simulink model "AttAndOrbitPropagator"  (R2017a)
settings: Solver=FixedStepAuto  StartTime=0.0  StopTime=24*3600  FixedStep=10  RelTol=1e-3  EnableMultiTasking=on
PreLoadFcn:
  | InitialiseJ2
values from neighbouring files (symbols this model uses):
  a = (mu/(n*2*pi/(24*3600))^2)^(1/3)    [InitialiseJ2.m]
  e = L3(1,5)/1e7    [InitialiseJ2.m]
  h = (mu*rp*(1 + e))^0.5    [InitialiseJ2.m]
  i = L3(1,3)    [InitialiseJ2.m]
  J2 = 0.0010836    [InitialiseJ2.m]
  mu = 398600.4415    [InitialiseJ2.m]
  omega = L3(1,6)    [InitialiseJ2.m]
  R_earth = 6378.137    [InitialiseJ2.m]
  RAAN = L3(1,4)    [InitialiseJ2.m]
  T = 2*pi*sqrt(a^3/mu)    [InitialiseJ2.m]
  t0 = M/(2*pi)*T    [InitialiseJ2.m]
libraries: sharedtransform x4, vrlib x3
settings Model: PauseTimes=0  NumberOfSteps=10  SnapshotBufferSize=10000  SnapshotInterval=1  Creator="TEAM  STUDSAT -2"  LastModifiedBy=Navaneet
settings OptimizationCC: LifeSpan=inf
settings DebuggingCC: SFUnexpectedBacktrackingDiag=warning  SFNoUnconditionalDefaultTransitionDiag=warning  SFExecutionAtInitializationDiag=none
settings GRTTargetCC: TargetLangStandard=C89/C90 (ANSI)  GeneratePreprocessorConditionals=Disable all
settings ConfigComp: CovMetricSettings=dw  CovHtmlReporting=on  CovSaveCumulativeToWorkspaceVar=on  CovSaveSingleToWorkspaceVar=on  CovExternalEMLEnable=off

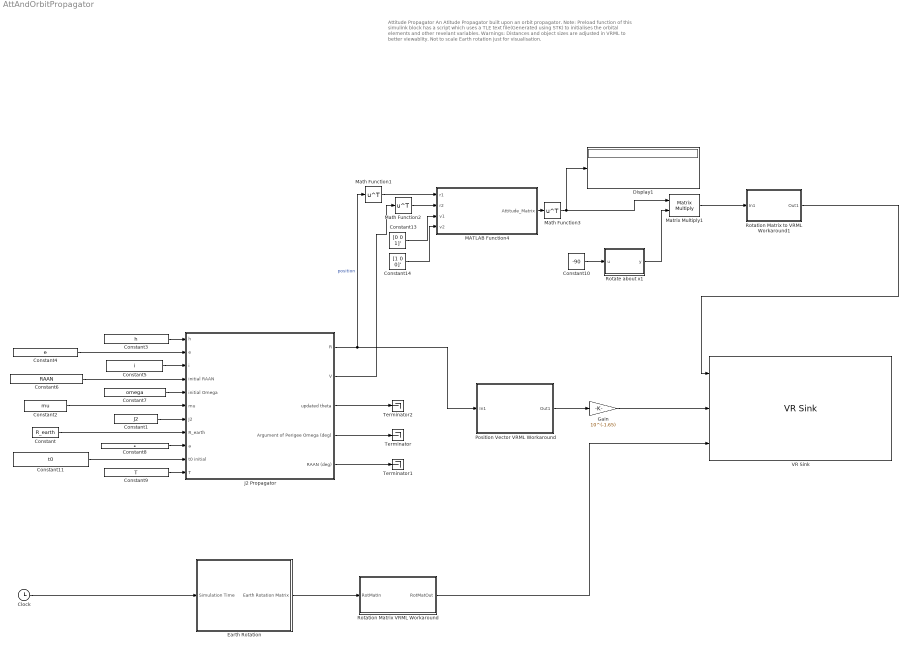
== system AttAndOrbitPropagator ==
  note: Attitude Propagator
      | An Atitude Propagator built upon an orbit propagator.
      |
      | Note:
      | Preload function of this simulink block has a script which uses a TLE text file(Generated using STK) to initialises the orbital elements and other revelant variables.
      |
      | Warnings:
      | Distances and object sizes are adjusted in VRML to better viewablity. Not to scale
      | Earth rotation just for visualisation.
  Clock : Clock
  Constant : Constant  Value=R_earth
  Constant1 : Constant  Value=J2
  Constant10 : Constant  Value=-90
  Constant11 : Constant  Value=t0
  Constant13 : Constant  Value=[0 0 1]'  VectorParams1D=off
  Constant14 : Constant  Value=[1 0 0]'  VectorParams1D=off
  Constant2 : Constant  Value=mu
  Constant3 : Constant  Value=h
  Constant4 : Constant  Value=e
  Constant5 : Constant  Value=i
  Constant6 : Constant  Value=RAAN
  Constant7 : Constant  Value=omega
  Constant8 : Constant  Value=a
  Constant9 : Constant  Value=T
  Display1 : Display
  Earth Rotation : Subsystem
  Gain : Gain  Gain=10^(-1.65)
  J2 Propagator : Subsystem
  MATLAB Function4 : MATLAB Function  TreatAsAtomicUnit=on
  Math Function1 : Math  Operator=transpose  SaturateOnIntegerOverflow=on
  Math Function2 : Math  Operator=transpose  SaturateOnIntegerOverflow=on
  Math Function3 : Math  Operator=transpose  SaturateOnIntegerOverflow=on
  Matrix Multiply1 : Product  Multiplication=Matrix(*)
  Position Vector VRML Workaround : Subsystem
  Rotate about x1 : MATLAB Function  TreatAsAtomicUnit=on
  Rotation Matrix VRML Workaround : Subsystem
  Rotation Matrix to VRML Workaround1 : Subsystem
  Terminator : Terminator
  Terminator1 : Terminator
  Terminator2 : Terminator
  VR Sink : vrlib/VR Sink  InstantiateOnLoad=on  SampleTime=-1  ViewEnable=on  RemoteChange=off  RemoteView=off  FieldsWritten=Satellite.rotation.4.1.1.double#Satellite.translation.3.1.1.double#Earth.rotation.4.1.1.double  WorldFileName=earthSatSys_Ideal.WRL  AutoView=off  VideoDimensions=[]  AllowVariableSize=off  FigureProperties="{'Position', 'Name', 'Viewpoint', 'CameraBound', 'CameraDirection', 'CameraPosition', 'CameraUpVector', 'ZoomFactor', 'Antialiasing', 'Headlight', 'Lighting', 'NavPanel', 'Sound', 'StatusBar', 'Stereo3D', 'Stereo3DCameraOffset', 'Stereo3DHIT', 'ToolBar', 'Textures', 'Transparency', 'Triad', 'Wireframe', 'NavZones', 'NavMode', 'NavSpeed', 'CaptureFileFormat', 'CaptureFileName', 'Record2DCompressMethod', 'Record2DCompressQuality', 'Record2D', 'Record2DFileName', 'Record2DFPS'; [2.5700000000000000e+02   2.3400000000000000e+02   5.7600000000000000e+02   3.5000000000000000e+02], '', 'Front_View', 'on', [0.0000000000000000e+00   0.0000000000000000e+00  -1.0000000000000000e+00], [0.0000000000000000e+00   0.0000000000000000e+00   0.0000000000000000e+00], [0.0000000000000000e+00   1.0000000000000000e+00   0.0000000000000000e+00], [1.0000000000000000e+00], 'on', 'on', 'on', 'halfbar', 'on', 'on', 'off', [1.0000000149011612e-01], [0.0000000000000000e+00], 'on', 'on', 'on', 'none', 'off', 'off', 'fly', 'normal', 'tif', '%f_anim_%n.tif', 'auto', [7.5000000000000000e+01], 'off', '%f_anim_%n.avi', 'auto'}"
      settings: SourceProductBaseCode=VR
  wires:
  Constant/1 -> J2 Propagator/8(R_earth)
  Constant1/1 -> J2 Propagator/7(J2)
  Constant2/1 -> J2 Propagator/6(mu)
  Constant3/1 -> J2 Propagator/1(h)
  Constant4/1 -> J2 Propagator/2(e)
  Constant5/1 -> J2 Propagator/3(i)
  Constant6/1 -> J2 Propagator/4(initial RAAN)
  Constant8/1 -> J2 Propagator/9(a)
  Constant11/1 -> J2 Propagator/10(t0 initial)
  Constant9/1 -> J2 Propagator/11(T)
  Constant7/1 -> J2 Propagator/5(initial Omega)
  J2 Propagator/4(Argument of Perigee Omega (deg)) -> Terminator/1
  J2 Propagator/3(updated theta) -> Terminator2/1
  Earth Rotation/1(Earth Rotation Matrix) -> Rotation Matrix VRML Workaround/1(RotMatIn)
  Position Vector VRML Workaround/1(Out1) -> Gain/1
  J2 Propagator/5(RAAN (deg)) -> Terminator1/1
  Clock/1 -> Earth Rotation/1(Simulation Time)
  MATLAB Function4/1(Attitude_Matrix) -> Math Function3/1
  Constant10/1 -> Rotate about x1/1(u)
  J2 Propagator/2(V) -> Math Function2/1
  Matrix Multiply1/1 -> Rotation Matrix to VRML Workaround1/1(In1)
  Math Function3/1 -> Matrix Multiply1/1, Display1/1
  ? -> ?
  Rotate about x1/1(y) -> Matrix Multiply1/2
  Rotation Matrix to VRML Workaround1/1(Out1) -> VR Sink/1
  J2 Propagator/1(R) -> Math Function1/1, Position Vector VRML Workaround/1(In1)  "position"
  Constant14/1 -> MATLAB Function4/4(v2)
  Constant13/1 -> MATLAB Function4/3(v1)
  Math Function2/1 -> MATLAB Function4/2(r2)
  Math Function1/1 -> MATLAB Function4/1(r1)
  Gain/1 -> VR Sink/2
  Rotation Matrix VRML Workaround/1(RotMatOut) -> VR Sink/3

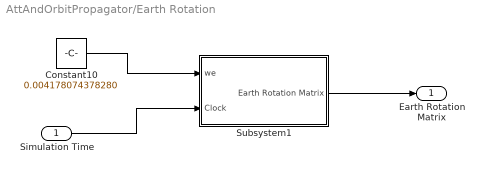
== system AttAndOrbitPropagator/Earth Rotation ==
  Simulation Time : Inport
  Constant10 : Constant  Value=0.004178074378280
  Subsystem1 : Subsystem
  Earth Rotation Matrix : Outport
  wires:
  Constant10/1 -> Subsystem1/1(we)
  Simulation Time/1 -> Subsystem1/2(Clock)
  Subsystem1/1(Earth Rotation Matrix) -> Earth Rotation Matrix/1

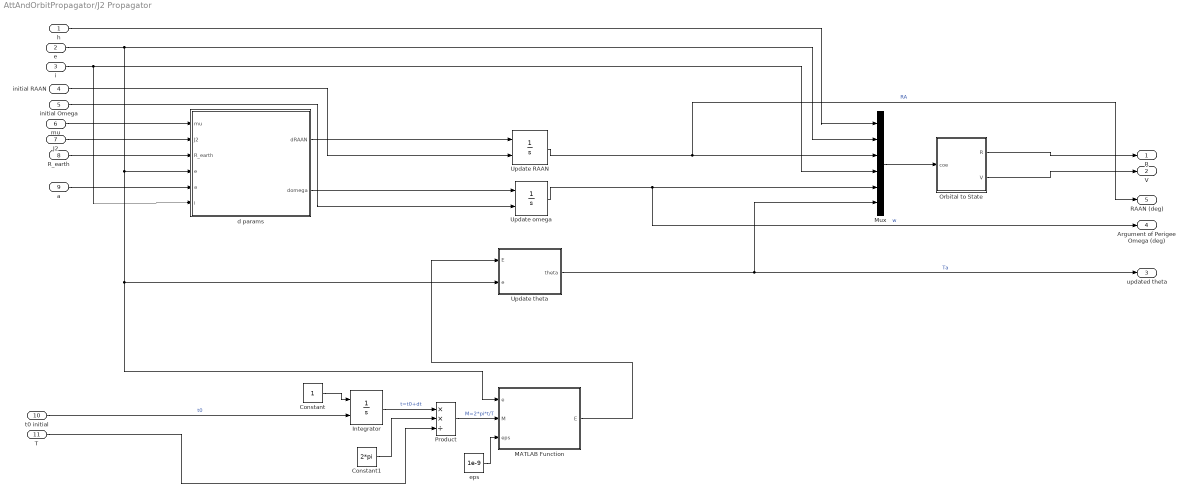
== system AttAndOrbitPropagator/J2 Propagator ==
  h : Inport
  e : Inport  Port=2
  i : Inport  Port=3
  initial RAAN : Inport  Port=4
  initial Omega : Inport  Port=5
  mu : Inport  Port=6
  J2 : Inport  Port=7
  R_earth : Inport  Port=8
  a : Inport  Port=9
  t0 initial : Inport  Port=10
  T : Inport  Port=11
  Constant : Constant
  Constant1 : Constant  Value=2*pi
  Integrator : Integrator  InitialConditionSource=external
  MATLAB Function : MATLAB Function  TreatAsAtomicUnit=on
  Mux : Mux  Inputs=6
  Orbital to State : MATLAB Function  TreatAsAtomicUnit=on
  Product : Product  Inputs=**/
  Update RAAN : Integrator  InitialConditionSource=external
  Update omega : Integrator  InitialConditionSource=external
  Update theta : MATLAB Function  TreatAsAtomicUnit=on
  d params : MATLAB Function  TreatAsAtomicUnit=on
  eps : Constant  Value=1e-9
  R : Outport
  V : Outport  Port=2
  updated theta : Outport  Port=3
  Argument of Perigee Omega (deg) : Outport  Port=4
  RAAN (deg) : Outport  Port=5
  wires:
  eps/1 -> MATLAB Function/3(eps)
  mu/1 -> d params/1(mu)
  a/1 -> d params/5(a)
  J2/1 -> d params/2(J2)
  R_earth/1 -> d params/3(R_earth)
  MATLAB Function/1(E) -> Update theta/1(E)
  t0 initial/1 -> Integrator/2  "t0"
  Constant/1 -> Integrator/1
  Integrator/1 -> Product/1  "t=t0+dt"
  T/1 -> Product/3
  Constant1/1 -> Product/2
  d params/1(dRAAN) -> Update RAAN/1
  initial RAAN/1 -> Update RAAN/2
  d params/2(domega) -> Update omega/1
  initial Omega/1 -> Update omega/2
  h/1 -> Mux/1
  i/1 -> d params/6(i), Mux/4
  Mux/1 -> Orbital to State/1(coe)
  Product/1 -> MATLAB Function/2(M)  "M=2*pi*t/T"
  Update omega/1 -> Argument of Perigee Omega (deg)/1, Mux/5  "w"
  Update theta/1(theta) -> Mux/6, updated theta/1  "Ta"
  Update RAAN/1 -> RAAN (deg)/1, Mux/3  "RA"
  e/1 -> MATLAB Function/1(e), Update theta/2(e), d params/4(e), Mux/2
  Orbital to State/1(R) -> R/1
  Orbital to State/2(V) -> V/1

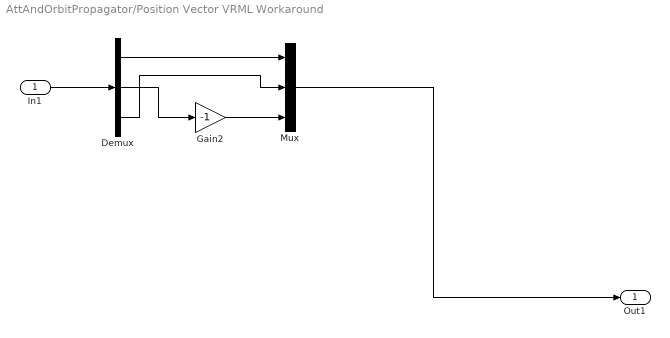
== system AttAndOrbitPropagator/Position Vector VRML Workaround ==
  In1 : Inport
  Demux : Demux  Outputs=3
  Gain2 : Gain  Gain=-1
  Mux : Mux  Inputs=3
  Out1 : Outport
  wires:
  Demux/1 -> Mux/1
  Demux/2 -> Gain2/1
  Demux/3 -> Mux/2
  Mux/1 -> Out1/1
  Gain2/1 -> Mux/3
  In1/1 -> Demux/1

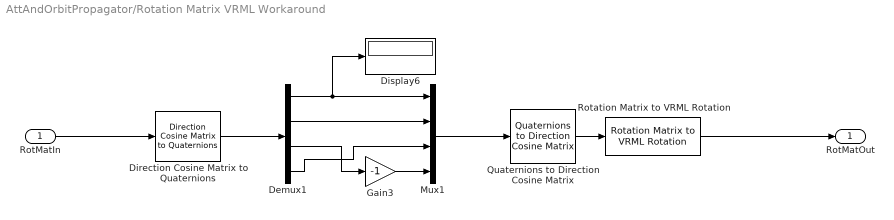
== system AttAndOrbitPropagator/Rotation Matrix VRML Workaround ==
  RotMatIn : Inport
  Demux1 : Demux
  Direction Cosine Matrix to Quaternions : sharedtransform/Direction Cosine Matrix  to Quaternions
  Display6 : Display
  Gain3 : Gain  Gain=-1
  Mux1 : Mux
  Quaternions to Direction Cosine Matrix : sharedtransform/Quaternions to  Direction Cosine Matrix
  Rotation Matrix to VRML Rotation : vrlib/Utilities/Rotation Matrix to VRML Rotation  maxzero=1e-12
      settings: SourceProductName=Simulink 3D Animation  SourceProductBaseCode=VR
  RotMatOut : Outport
  wires:
  RotMatIn/1 -> Direction Cosine Matrix to Quaternions/1
  Direction Cosine Matrix to Quaternions/1 -> Demux1/1
  Demux1/3 -> Gain3/1
  Gain3/1 -> Mux1/4
  Demux1/4 -> Mux1/3
  Demux1/2 -> Mux1/2
  Demux1/1 -> Display6/1, Mux1/1
  Mux1/1 -> Quaternions to Direction Cosine Matrix/1
  Quaternions to Direction Cosine Matrix/1 -> Rotation Matrix to VRML Rotation/1
  Rotation Matrix to VRML Rotation/1 -> RotMatOut/1

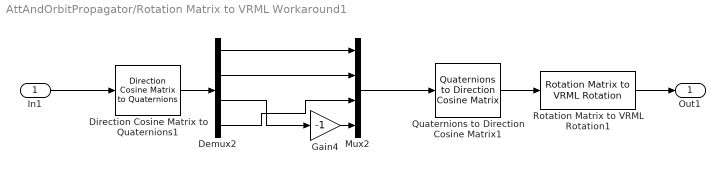
== system AttAndOrbitPropagator/Rotation Matrix to VRML Workaround1 ==
  In1 : Inport
  Demux2 : Demux
  Direction Cosine Matrix to Quaternions1 : sharedtransform/Direction Cosine Matrix  to Quaternions
  Gain4 : Gain  Gain=-1
  Mux2 : Mux
  Quaternions to Direction Cosine Matrix1 : sharedtransform/Quaternions to  Direction Cosine Matrix
  Rotation Matrix to VRML Rotation1 : vrlib/Utilities/Rotation Matrix to VRML Rotation  maxzero=1e-12
      settings: SourceProductName=Simulink 3D Animation  SourceProductBaseCode=VR
  Out1 : Outport
  wires:
  Direction Cosine Matrix to Quaternions1/1 -> Demux2/1
  Rotation Matrix to VRML Rotation1/1 -> Out1/1
  Mux2/1 -> Quaternions to Direction Cosine Matrix1/1
  Demux2/4 -> Mux2/3
  Demux2/3 -> Gain4/1
  Gain4/1 -> Mux2/4
  Demux2/1 -> Mux2/1
  Demux2/2 -> Mux2/2
  Quaternions to Direction Cosine Matrix1/1 -> Rotation Matrix to VRML Rotation1/1
  In1/1 -> Direction Cosine Matrix to Quaternions1/1

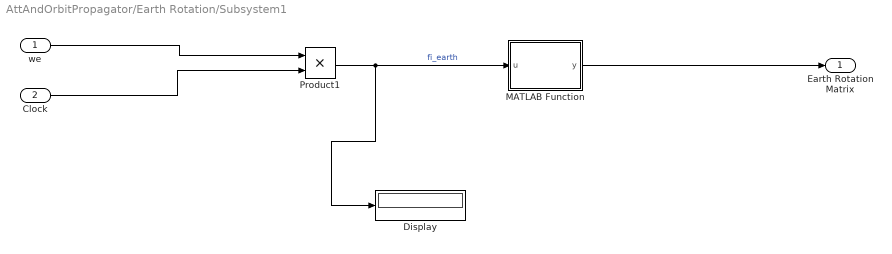
== system AttAndOrbitPropagator/Earth Rotation/Subsystem1 ==
  we : Inport
  Clock : Inport  Port=2
  Display : Display
  MATLAB Function : MATLAB Function  TreatAsAtomicUnit=on
  Product1 : Product
  Earth Rotation Matrix : Outport
  wires:
  Clock/1 -> Product1/2
  we/1 -> Product1/1
  Product1/1 -> MATLAB Function/1(u), Display/1  "fi_earth"
  MATLAB Function/1(y) -> Earth Rotation Matrix/1

== matlab function AttAndOrbitPropagator/Earth Rotation/Subsystem1/MATLAB Function ==
  data: u input; y output
function y = fcn(u)
%#codegen

y =rotz(u);

== matlab function AttAndOrbitPropagator/J2 Propagator/d params ==
  data: mu input; dRAAN output; J2 input; R_earth input; e input; a input; i input; domega output
function [dRAAN, domega]=dparams(mu,J2, R_earth,e,a,i)

dRAAN = -(1.5*mu^0.5*J2*R_earth^2/((1-e^2)*a^3.5))*cosd(i)*180/pi;
domega = dRAAN*(2.5*sind(i)^2 - 2)/cosd(i);
end

== matlab function AttAndOrbitPropagator/J2 Propagator/MATLAB Function ==
  data: e input; M input; E output; eps input
function E = keplerEq(e,M,eps)
En  = M;
Ens = En - (En-e*sin(En)- M)/(1 - e*cos(En));
while ( abs(Ens-En) > eps )
    En = Ens;
    Ens = En - (En - e*sin(En) - M)/(1 - e*cos(En));
end;
E = Ens;
end

== matlab function AttAndOrbitPropagator/J2 Propagator/Update theta ==
  data: E input; theta output; e input
function theta = updateTheta(E,e)
theta=2*atan(tan(E/2)*((1+e)/(1-e))^0.5)*180/pi;

end

== matlab function AttAndOrbitPropagator/J2 Propagator/Orbital to State ==
  data: coe input; R output size=[1 3]; V output size=[1 3]
function [R, V] = Orbital2State(coe)

% ˜˜˜˜˜˜˜˜˜˜˜˜˜˜˜˜˜˜˜˜˜˜˜˜˜˜˜˜˜˜˜˜˜˜
% This function computes the state vector (r,v) from the
% classical orbital elements (coe).
%
% mu - gravitational parameter (kmˆ3; sˆ2)
% coe - orbital elements [h e RA incl w TA]
% where
% h = angular momentum (kmˆ2/s)
% e = eccentricity
% RA = right ascension of the ascending node (rad)
% incl = inclination of the orbit (rad)
% w = argument of perigee (rad)
% TA = true anomaly (rad)
% R3_w - Rotation matrix about the z-axis through the angle w
% R1_i - Rotation matrix about the x-axis through the angle i
% R3_W - Rotation matrix about the z-axis through the angle RA
% Q_pX - Matrix of the transformation from perifocal to
% geocentric equatorial frame
% rp - position vector in the perifocal frame (km)
% vp - velocity vector in the perifocal frame (km/s)
% r - position vector in the geocentric equatorial frame
% (km)
% v - velocity vector in the geocentric equatorial frame
% (km/s)
%
% User M-functions required: none
% ------------------------------------------------------------
mu    = 398600; 
h = coe(1);
e = coe(2);
RA = coe(3)*pi/180;
incl = coe(4)*pi/180;
w = coe(5)*pi/180;
TA = coe(6)*pi/180;
%...Equations 4.37 and 4.38 (rp and vp are column vectors):
rp = (h^2/mu) * (1/(1 + e*cos(TA))) * (cos(TA)*[1;0;0] ...
+ sin(TA)*[0;1;0]);
vp = (mu/h) * (-sin(TA)*[1;0;0] + (e + cos(TA))*[0;1;0]);
%...Equation 4.39:
R3_W = [ cos(RA) sin(RA) 0
-sin(RA) cos(RA) 0
0 0 1];
%...Equation 4.40:
R1_i = [1 0 0
0 cos(incl) sin(incl)
0 -sin(incl) cos(incl)];
%...Equation 4.41:
R3_w = [ cos(w) sin(w) 0
-sin(w) cos(w) 0
0 0 1];
%...Equation 4.44:
Q_pX = R3_W'*R1_i'*R3_w';
%...Equations 4.46 (r and v are column vectors):
r = Q_pX*rp;
v = Q_pX*vp;
%...Convert r and v into row vectors:
R = r';
V = v';
% ˜˜˜˜˜˜˜˜˜˜˜˜˜˜˜˜˜˜˜˜˜˜˜˜˜˜˜˜˜˜˜˜˜˜˜˜˜˜˜˜˜˜˜˜˜˜˜˜˜˜˜˜˜˜˜˜˜˜˜˜

== matlab function AttAndOrbitPropagator/Rotate about x1 ==
  data: u input; y output
function y = fcn(u)
%#codegen

y =rotx(u);

== matlab function AttAndOrbitPropagator/MATLAB Function4 ==
  data: r1 input; Attitude_Matrix output; r2 input; v1 input; v2 input
function Attitude_Matrix=Triad(r1,r2,v1,v2)
%This function generates an attitude matrix two reference and two measured
%vectors.

%Tackle Anomaly 1: when both vectors are same cross product is invalid. So,
if r1==r2
    r2(1)=r2(1)+0.0000000000000001;
end
if v1==v2
    v2(1)=v2(1)+0.0000000000000001;
end
%Calculate body tirad
t1b=v1./norm(v1);
t2b=cross(t1b,v2)./norm(cross(t1b,v2));
t3b=cross(t1b,t2b)./norm(cross(t1b,t2b));

%Calculate reference tirad
t1r=r1./norm(r1);
t2r=cross(t1r,r2)./norm(cross(t1r,r2));
t3r=cross(t1r,t2r)./norm(cross(t1r,t2r));

%Calculate attituce matrix
Attitude_Matrix= t1b*(t1r.') + t2b*(t2r.') + t3b*(t3r.');
